simulink model "Comp_FDC_main"  (R2021b)
settings: Solver=FixedStepDiscrete  StartTime=0.0  StopTime=10.0  RelTol=1e-3  EnableMultiTasking=on
undefined symbols (not defined in the file or in its folder): D1, P
settings Model: DataDictionary=APPTypes.sldd  Creator=FVT23118  LastModifiedBy=FVT23118
settings SolverCC: AutoInsertRateTranBlk=on
settings DataIOCC: SaveFormat=StructureWithTime
settings OptimizationCC: DefaultParameterBehavior=Inlined  EnhancedBackFolding=on  PassReuseOutputArgsAs=Individual arguments  ZeroExternalMemoryAtStartup=off  ZeroInternalMemoryAtStartup=off  OptimizeBlockOrder=speed  DifferentSizesBufferReuse=on  OptimizationCustomize=off  EfficientTunableParamExpr=on
settings DebuggingCC: ParameterTunabilityLossMsg=error
settings ModelReferenceCC: ModelReferenceNumInstancesAllowed=Single
settings SFSimCC: MATLABDynamicMemAlloc=off
settings RTWCC: Description=AUTOSAR  SystemTargetFile=autosar.tlc  GenCodeOnly=on  TemplateMakefile=ert_default_tmf
settings CodeAppCC: ForceParamTrailComments=on  IgnoreCustomStorageClasses=off  OperatorAnnotations=on  SimulinkDataObjDesc=on  SFDataObjDesc=on  InsertBlockDesc=on
settings STFCustomTargetCC: TargetLangStandard=C99 (ISO)  MultiwordLength=256  ParMdlRefBuildCompliant=on  CompOptLevelCompliant=on  IncludeMdlTerminateFcn=off  CombineOutputUpdateFcns=on  SuppressErrorStatus=on  ERTCustomFileBanners=on  SupportNonFinite=off  SupportComplex=off  SupportContinuousTime=off  SupportNonInlinedSFcns=off  RemoveResetFunc=on  MATLABClassNameForMDSCustomization=Simulink.SoftwareTarget.ERTCustomization  AutosarCompliant=on  GRTInterface=off  UseToolchainInfoCompliant=on  LookupTableObjectStructAxisOrder=2,1,3,4,...  LUTObjectStructOrderEvenSpacing=Size,Table,Breakpoints  SystemTargetFile=autosar.tlc
settings ERTTargetCC: TargetLangStandard=C99 (ISO)  ConcurrentExecutionCompliant=off  IncludeMdlTerminateFcn=off  SuppressErrorStatus=on  SupportNonFinite=off  SupportComplex=off  ModelStepFunctionPrototypeControlCompliant=off  CPPClassGenCompliant=off  AutosarCompliant=on  LookupTableObjectStructAxisOrder=2,1,3,4,...  LUTObjectStructOrderEvenSpacing=Size,Table,Breakpoints  InlinedParameterPlacement=NonHierarchical  ERTCustomFileTemplate=example_file_process.tlc

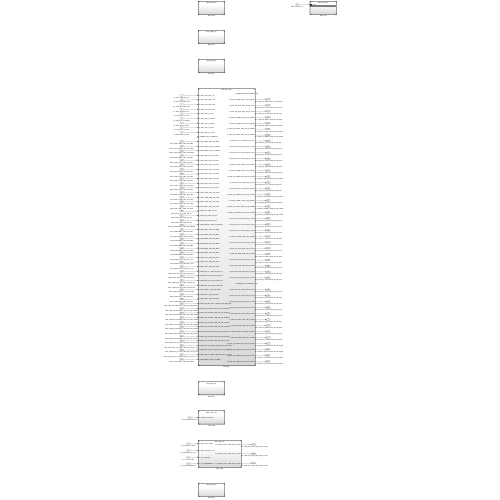
[thumbnail: Simulink's stored preview of the top-level diagram]
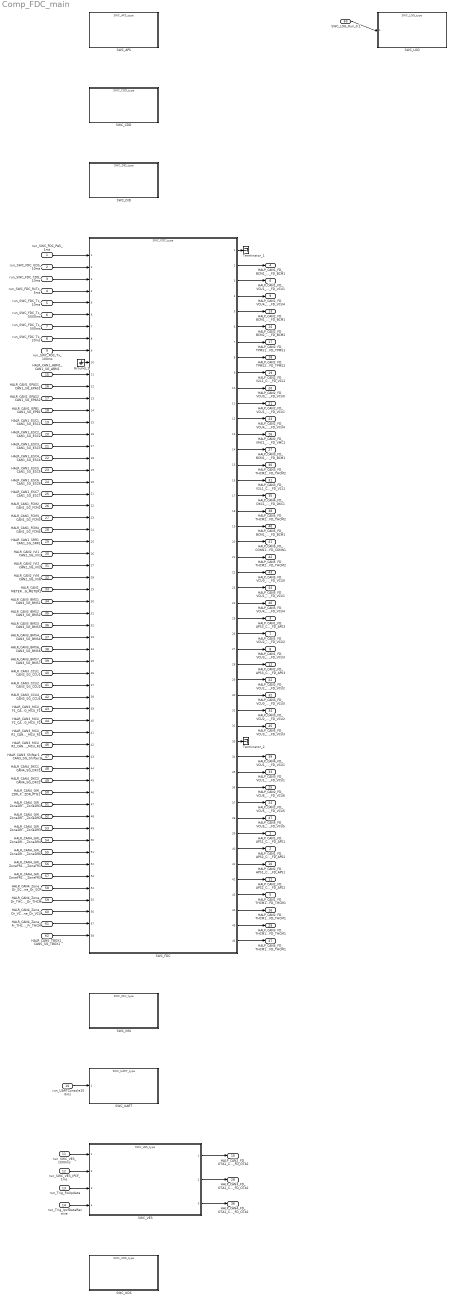
== system Comp_FDC_main ==
  run_SWC_FDC_PAS_1ms : Inport  SampleTime=0.001  OutputFunctionCall=on
  run_SWC_FDC_UDS_10ms : Inport  Port=2  SampleTime=0.01  OutputFunctionCall=on
  run_SWC_FDC_CDD_10ms : Inport  Port=3  SampleTime=0.01  OutputFunctionCall=on
  run_SWC_FDC_RxTx_5ms : Inport  Port=4  SampleTime=0.005  OutputFunctionCall=on
  run_SWC_FDC_Tx_10ms : Inport  Port=5  SampleTime=0.01  OutputFunctionCall=on
  run_SWC_FDC_Tx_5000ms : Inport  Port=6  SampleTime=5  OutputFunctionCall=on
  run_SWC_FDC_Tx_500ms : Inport  Port=7  SampleTime=0.5  OutputFunctionCall=on
  run_SWC_FDC_Tx_20ms : Inport  Port=8  SampleTime=0.02  OutputFunctionCall=on
  run_SWC_FDC_Tx_100ms : Inport  Port=9  SampleTime=0.1  OutputFunctionCall=on
  run_UARTConsole100ms : Inport  Port=10  SampleTime=0.1  OutputFunctionCall=on
  run_SWC_VES_1000ms : Inport  Port=11  SampleTime=1  OutputFunctionCall=on
  run_SWC_VES_IPCF_1ms : Inport  Port=12  SampleTime=0.001  OutputFunctionCall=on
  run_Trig_FwUpdate : Inport  Port=13  OutputFunctionCall=on
  run_Trig_IpcfDataReceive : Inport  Port=14  OutputFunctionCall=on
  HALR_CAN1_ABM1_CAN1_SG_ABM1 : Inport  Port=15  OutDataTypeStr=Bus: DT_CAN1_SG_ABM1  PortDimensions=1  BusOutputAsStruct=on
  HALR_CAN1_EPAS1_CAN1_SG_EPAS1 : Inport  Port=16  OutDataTypeStr=Bus: DT_CAN1_SG_EPAS1  PortDimensions=1  BusOutputAsStruct=on
  HALR_CAN1_EPAS2_CAN1_SG_EPAS2 : Inport  Port=17  OutDataTypeStr=Bus: DT_CAN1_SG_EPAS2  PortDimensions=1  BusOutputAsStruct=on
  HALR_CAN1_EPB1_CAN1_SG_EPB1 : Inport  Port=18  OutDataTypeStr=Bus: DT_CAN1_SG_EPB1  PortDimensions=1  BusOutputAsStruct=on
  HALR_CAN1_ESC1_CAN1_SG_ESC1 : Inport  Port=19  OutDataTypeStr=Bus: DT_CAN1_SG_ESC1  PortDimensions=1  BusOutputAsStruct=on
  HALR_CAN1_ESC2_CAN1_SG_ESC2 : Inport  Port=20  OutDataTypeStr=Bus: DT_CAN1_SG_ESC2  PortDimensions=1  BusOutputAsStruct=on
  HALR_CAN1_ESC3_CAN1_SG_ESC3 : Inport  Port=21  OutDataTypeStr=Bus: DT_CAN1_SG_ESC3  PortDimensions=1  BusOutputAsStruct=on
  HALR_CAN1_ESC4_CAN1_SG_ESC4 : Inport  Port=22  OutDataTypeStr=Bus: DT_CAN1_SG_ESC4  PortDimensions=1  BusOutputAsStruct=on
  HALR_CAN1_ESC5_CAN1_SG_ESC5 : Inport  Port=23  OutDataTypeStr=Bus: DT_CAN1_SG_ESC5  PortDimensions=1  BusOutputAsStruct=on
  HALR_CAN1_ESC6_CAN1_SG_ESC6 : Inport  Port=24  OutDataTypeStr=Bus: DT_CAN1_SG_ESC6  PortDimensions=1  BusOutputAsStruct=on
  HALR_CAN1_ESC7_CAN1_SG_ESC7 : Inport  Port=25  OutDataTypeStr=Bus: DT_CAN1_SG_ESC7  PortDimensions=1  BusOutputAsStruct=on
  HALR_CAN1_FCM2_CAN1_SG_FCM2 : Inport  Port=26  OutDataTypeStr=Bus: DT_CAN1_SG_FCM2  PortDimensions=1  BusOutputAsStruct=on
  HALR_CAN1_FCM3_CAN1_SG_FCM3 : Inport  Port=27  OutDataTypeStr=Bus: DT_CAN1_SG_FCM3  PortDimensions=1  BusOutputAsStruct=on
  HALR_CAN1_FCM4_CAN1_SG_FCM4 : Inport  Port=28  OutDataTypeStr=Bus: DT_CAN1_SG_FCM4  PortDimensions=1  BusOutputAsStruct=on
  HALR_CAN1_SRR1_CAN1_SG_SRR1 : Inport  Port=29  OutDataTypeStr=Bus: DT_CAN1_SG_SRR1  PortDimensions=1  BusOutputAsStruct=on
  HALR_CAN2_IVI1_CAN2_SG_IVI1 : Inport  Port=30  OutDataTypeStr=Bus: DT_CAN2_SG_IVI1  PortDimensions=1  BusOutputAsStruct=on
  HALR_CAN2_IVI2_CAN2_SG_IVI2 : Inport  Port=31  OutDataTypeStr=Bus: DT_CAN2_SG_IVI2  PortDimensions=1  BusOutputAsStruct=on
  HALR_CAN2_IVI6_CAN2_SG_IVI6 : Inport  Port=32  OutDataTypeStr=Bus: DT_CAN2_SG_IVI6  PortDimensions=1  BusOutputAsStruct=on
  HALR_CAN2_METER1_CAN2_SG_METER1 : Inport  Port=33  OutDataTypeStr=Bus: DT_CAN2_SG_METER1  PortDimensions=1  BusOutputAsStruct=on
  HALR_CAN3_BMS1_CAN3_SG_BMS1 : Inport  Port=34  OutDataTypeStr=Bus: DT_CAN3_SG_BMS1  PortDimensions=1  BusOutputAsStruct=on
  HALR_CAN3_BMS2_CAN3_SG_BMS2 : Inport  Port=35  OutDataTypeStr=Bus: DT_CAN3_SG_BMS2  PortDimensions=1  BusOutputAsStruct=on
  HALR_CAN3_BMS3_CAN3_SG_BMS3 : Inport  Port=36  OutDataTypeStr=Bus: DT_CAN3_SG_BMS3  PortDimensions=1  BusOutputAsStruct=on
  HALR_CAN3_BMS4_CAN3_SG_BMS4 : Inport  Port=37  OutDataTypeStr=Bus: DT_CAN3_SG_BMS4  PortDimensions=1  BusOutputAsStruct=on
  HALR_CAN3_BMS6_CAN3_SG_BMS6 : Inport  Port=38  OutDataTypeStr=Bus: DT_CAN3_SG_BMS6  PortDimensions=1  BusOutputAsStruct=on
  HALR_CAN3_BMS7_CAN3_SG_BMS7 : Inport  Port=39  OutDataTypeStr=Bus: DT_CAN3_SG_BMS7  PortDimensions=1  BusOutputAsStruct=on
  HALR_CAN3_CCU1_CAN3_SG_CCU1 : Inport  Port=40  OutDataTypeStr=Bus: DT_CAN3_SG_CCU1  PortDimensions=1  BusOutputAsStruct=on
  HALR_CAN3_CCU2_CAN3_SG_CCU2 : Inport  Port=41  OutDataTypeStr=Bus: DT_CAN3_SG_CCU2  PortDimensions=1  BusOutputAsStruct=on
  HALR_CAN3_CCU4_CAN3_SG_CCU4 : Inport  Port=42  OutDataTypeStr=Bus: DT_CAN3_SG_CCU4  PortDimensions=1  BusOutputAsStruct=on
  HALR_CAN3_MCU_F1_CAN3_SG_MCU_F1 : Inport  Port=43  OutDataTypeStr=Bus: DT_CAN3_SG_MCU_F1  PortDimensions=1  BusOutputAsStruct=on
  HALR_CAN3_MCU_F2_CAN3_SG_MCU_F2 : Inport  Port=44  OutDataTypeStr=Bus: DT_CAN3_SG_MCU_F2  PortDimensions=1  BusOutputAsStruct=on
  HALR_CAN3_MCU_R1_CAN3_SG_MCU_R1 : Inport  Port=45  OutDataTypeStr=Bus: DT_CAN3_SG_MCU_R1  PortDimensions=1  BusOutputAsStruct=on
  HALR_CAN3_MCU_R2_CAN3_SG_MCU_R2 : Inport  Port=46  OutDataTypeStr=Bus: DT_CAN3_SG_MCU_R2  PortDimensions=1  BusOutputAsStruct=on
  HALR_CAN3_Shifter1_CAN3_SG_Shifter1 : Inport  Port=47  OutDataTypeStr=Bus: DT_CAN3_SG_Shifter1  PortDimensions=1  BusOutputAsStruct=on
  HALR_CAN4_DKC1_CAN4_SG_DKC1 : Inport  Port=48  OutDataTypeStr=Bus: DT_CAN4_SG_DKC1  PortDimensions=1  BusOutputAsStruct=on
  HALR_CAN4_DKC2_CAN4_SG_DKC2 : Inport  Port=49  OutDataTypeStr=Bus: DT_CAN4_SG_DKC2  PortDimensions=1  BusOutputAsStruct=on
  HALR_CAN4_GW_ZDR_PTG1_CAN4_SG_GW_ZDR_PTG1 : Inport  Port=50  OutDataTypeStr=Bus: DT_CAN4_SG_GW_ZDR_PTG1  PortDimensions=1  BusOutputAsStruct=on
  HALR_CAN4_GW_ZoneDR1_CAN4_SG_GW_ZoneDR1 : Inport  Port=51  OutDataTypeStr=Bus: DT_CAN4_SG_GW_ZoneDR1  PortDimensions=1  BusOutputAsStruct=on
  HALR_CAN4_GW_ZoneDR2_CAN4_SG_GW_ZoneDR2 : Inport  Port=52  OutDataTypeStr=Bus: DT_CAN4_SG_GW_ZoneDR2  PortDimensions=1  BusOutputAsStruct=on
  HALR_CAN4_GW_ZoneDR3_CAN4_SG_GW_ZoneDR3 : Inport  Port=53  OutDataTypeStr=Bus: DT_CAN4_SG_GW_ZoneDR3  PortDimensions=1  BusOutputAsStruct=on
  HALR_CAN4_GW_ZoneDR4_CAN4_SG_GW_ZoneDR4 : Inport  Port=54  OutDataTypeStr=Bus: DT_CAN4_SG_GW_ZoneDR4  PortDimensions=1  BusOutputAsStruct=on
  HALR_CAN4_GW_ZoneDR6_CAN4_SG_GW_ZoneDR6 : Inport  Port=55  OutDataTypeStr=Bus: DT_CAN4_SG_GW_ZoneDR6  PortDimensions=1  BusOutputAsStruct=on
  HALR_CAN4_GW_ZoneFR1_CAN4_SG_GW_ZoneFR1 : Inport  Port=56  OutDataTypeStr=Bus: DT_CAN4_SG_GW_ZoneFR1  PortDimensions=1  BusOutputAsStruct=on
  HALR_CAN4_GW_ZoneFR2_CAN4_SG_GW_ZoneFR2 : Inport  Port=57  OutDataTypeStr=Bus: DT_CAN4_SG_GW_ZoneFR2  PortDimensions=1  BusOutputAsStruct=on
  HALR_CAN4_Zone_Dr_SCP_CAN4_SG_Zone_Dr_SCP : Inport  Port=58  OutDataTypeStr=Bus: DT_CAN4_SG_Zone_Dr_SCP  PortDimensions=1  BusOutputAsStruct=on
  HALR_CAN4_Zone_Dr_THCM_CAN4_SG_Zone_Dr_THCM : Inport  Port=59  OutDataTypeStr=Bus: DT_CAN4_SG_Zone_Dr_THCM  PortDimensions=1  BusOutputAsStruct=on
  HALR_CAN4_Zone_Dr_VCU_CAN4_SG_Zone_Dr_VCU : Inport  Port=60  OutDataTypeStr=Bus: DT_CAN4_SG_Zone_Dr_VCU  PortDimensions=1  BusOutputAsStruct=on
  HALR_CAN4_Zone_Fr_THCM_CAN4_SG_Zone_Fr_THCM : Inport  Port=61  OutDataTypeStr=Bus: DT_CAN4_SG_Zone_Fr_THCM  PortDimensions=1  BusOutputAsStruct=on
  HALR_CAN5_TBOX1_CAN5_SG_TBOX1 : Inport  Port=62  OutDataTypeStr=Bus: DT_CAN5_SG_TBOX1  PortDimensions=1  BusOutputAsStruct=on
  SWC_LOG_Run_0.1 : Inport  Port=63  SampleTime=0.1  OutputFunctionCall=on
  Ground_1 : Ground
  SWC_APS : ModelReference  ModelNameDialog=SWC_APS_type  SimulationMode=Normal  ScheduleRates=on  ModelReferenceVersion=1.3
  SWC_CDD : ModelReference  ModelNameDialog=SWC_CDD_type  SimulationMode=Normal  ScheduleRates=on  ModelReferenceVersion=1.5
  SWC_DID : ModelReference  ModelNameDialog=SWC_DID_type  SimulationMode=Normal  ScheduleRates=on  ModelReferenceVersion=1.5
  SWC_FDC : ModelReference  ModelNameDialog=SWC_FDC_type  SimulationMode=Normal  ScheduleRates=on  ModelReferenceVersion=1.30
  SWC_IMU : ModelReference  ModelNameDialog=SWC_IMU_type  SimulationMode=Normal  ScheduleRates=on  ModelReferenceVersion=1.3
  SWC_LOG : ModelReference  ModelNameDialog=SWC_LOG_type  SimulationMode=Normal  ScheduleRates=on  PortDiscreteRates=[0.1]  CachedPortDiscreteRates=[0.1]  ModelEventPortInfo=P:D1[0.1][0][0]  ModelReferenceVersion=1.4
  SWC_UART : ModelReference  ModelNameDialog=SWC_UART_type  SimulationMode=Normal  ScheduleRates=on  ModelReferenceVersion=1.3
  SWC_UDS : ModelReference  ModelNameDialog=SWC_UDS_type  SimulationMode=Normal  ScheduleRates=on  ModelReferenceVersion=1.3
  SWC_VES : ModelReference  ModelNameDialog=SWC_VES_type  SimulationMode=Normal  ScheduleRates=on  ModelReferenceVersion=1.4
  Terminator_1 : Terminator
  Terminator_2 : Terminator
  HALP_CAN1_FD_APS1_CAN1_SG_FD_APS1 : Outport  OutDataTypeStr=Bus: DT_CAN1_SG_FD_APS1  PortDimensions=1  BusOutputAsStruct=on
  HALP_CAN1_FD_APS2_CAN1_SG_FD_APS2 : Outport  Port=2  OutDataTypeStr=Bus: DT_CAN1_SG_FD_APS2  PortDimensions=1  BusOutputAsStruct=on
  HALP_CAN1_FD_APS3_CAN1_SG_FD_APS3 : Outport  Port=3  OutDataTypeStr=Bus: DT_CAN1_SG_FD_APS3  PortDimensions=1  BusOutputAsStruct=on
  HALP_CAN1_FD_BCM1_CAN1_SG_FD_BCM1 : Outport  Port=4  OutDataTypeStr=Bus: DT_CAN1_SG_FD_BCM1  PortDimensions=1  BusOutputAsStruct=on
  HALP_CAN1_FD_THCM1_CAN1_SG_FD_THCM1 : Outport  Port=5  OutDataTypeStr=Bus: DT_CAN1_SG_FD_THCM1  PortDimensions=1  BusOutputAsStruct=on
  HALP_CAN1_FD_VCU1_CAN1_SG_FD_VCU1 : Outport  Port=6  OutDataTypeStr=Bus: DT_CAN1_SG_FD_VCU1  PortDimensions=1  BusOutputAsStruct=on
  HALP_CAN1_FD_VCU2_CAN1_SG_FD_VCU2 : Outport  Port=7  OutDataTypeStr=Bus: DT_CAN1_SG_FD_VCU2  PortDimensions=1  BusOutputAsStruct=on
  HALP_CAN1_FD_VCU3_CAN1_SG_FD_VCU3 : Outport  Port=8  OutDataTypeStr=Bus: DT_CAN1_SG_FD_VCU3  PortDimensions=1  BusOutputAsStruct=on
  HALP_CAN1_FD_VCU4_CAN1_SG_FD_VCU4 : Outport  Port=9  OutDataTypeStr=Bus: DT_CAN1_SG_FD_VCU4  PortDimensions=1  BusOutputAsStruct=on
  HALP_CAN2_FD_APS1_CAN2_SG_FD_APS1 : Outport  Port=10  OutDataTypeStr=Bus: DT_CAN2_SG_FD_APS1  PortDimensions=1  BusOutputAsStruct=on
  HALP_CAN2_FD_APS2_CAN2_SG_FD_APS2 : Outport  Port=11  OutDataTypeStr=Bus: DT_CAN2_SG_FD_APS2  PortDimensions=1  BusOutputAsStruct=on
  HALP_CAN2_FD_APS3_CAN2_SG_FD_APS3 : Outport  Port=12  OutDataTypeStr=Bus: DT_CAN2_SG_FD_APS3  PortDimensions=1  BusOutputAsStruct=on
  HALP_CAN2_FD_BCM1_CAN2_SG_FD_BCM1 : Outport  Port=13  OutDataTypeStr=Bus: DT_CAN2_SG_FD_BCM1  PortDimensions=1  BusOutputAsStruct=on
  HALP_CAN2_FD_BCM2_CAN2_SG_FD_BCM2 : Outport  Port=14  OutDataTypeStr=Bus: DT_CAN2_SG_FD_BCM2  PortDimensions=1  BusOutputAsStruct=on
  HALP_CAN2_FD_OTA1_CAN2_SG_FD_OTA1 : Outport  Port=15  OutDataTypeStr=Bus: DT_CAN2_SG_FD_OTA1  PortDimensions=1  BusOutputAsStruct=on
  HALP_CAN2_FD_THCM1_CAN2_SG_FD_THCM1 : Outport  Port=16  OutDataTypeStr=Bus: DT_CAN2_SG_FD_THCM1  PortDimensions=1  BusOutputAsStruct=on
  HALP_CAN2_FD_TPMS1_CAN2_SG_FD_TPMS1 : Outport  Port=17  OutDataTypeStr=Bus: DT_CAN2_SG_FD_TPMS1  PortDimensions=1  BusOutputAsStruct=on
  HALP_CAN2_FD_TPMS2_CAN2_SG_FD_TPMS2 : Outport  Port=18  OutDataTypeStr=Bus: DT_CAN2_SG_FD_TPMS2  PortDimensions=1  BusOutputAsStruct=on
  HALP_CAN2_FD_V2L1_CAN2_SG_FD_V2L1 : Outport  Port=19  OutDataTypeStr=Bus: DT_CAN2_SG_FD_V2L1  PortDimensions=1  BusOutputAsStruct=on
  HALP_CAN2_FD_VCU0_CAN2_SG_FD_VCU0 : Outport  Port=20  OutDataTypeStr=Bus: DT_CAN2_SG_FD_VCU0  PortDimensions=1  BusOutputAsStruct=on
  HALP_CAN2_FD_VCU1_CAN2_SG_FD_VCU1 : Outport  Port=21  OutDataTypeStr=Bus: DT_CAN2_SG_FD_VCU1  PortDimensions=1  BusOutputAsStruct=on
  HALP_CAN2_FD_VCU2_CAN2_SG_FD_VCU2 : Outport  Port=22  OutDataTypeStr=Bus: DT_CAN2_SG_FD_VCU2  PortDimensions=1  BusOutputAsStruct=on
  HALP_CAN2_FD_VCU4_CAN2_SG_FD_VCU4 : Outport  Port=23  OutDataTypeStr=Bus: DT_CAN2_SG_FD_VCU4  PortDimensions=1  BusOutputAsStruct=on
  HALP_CAN2_FD_VCU5_CAN2_SG_FD_VCU5 : Outport  Port=24  OutDataTypeStr=Bus: DT_CAN2_SG_FD_VCU5  PortDimensions=1  BusOutputAsStruct=on
  HALP_CAN2_FD_VCU6_CAN2_SG_FD_VCU6 : Outport  Port=25  OutDataTypeStr=Bus: DT_CAN2_SG_FD_VCU6  PortDimensions=1  BusOutputAsStruct=on
  HALP_CAN2_FD_VMC1_CAN2_SG_FD_VMC1 : Outport  Port=26  OutDataTypeStr=Bus: DT_CAN2_SG_FD_VMC1  PortDimensions=1  BusOutputAsStruct=on
  HALP_CAN3_FD_BCM1_CAN3_SG_FD_BCM1 : Outport  Port=27  OutDataTypeStr=Bus: DT_CAN3_SG_FD_BCM1  PortDimensions=1  BusOutputAsStruct=on
  HALP_CAN3_FD_OTA1_CAN3_SG_FD_OTA1 : Outport  Port=28  OutDataTypeStr=Bus: DT_CAN3_SG_FD_OTA1  PortDimensions=1  BusOutputAsStruct=on
  HALP_CAN3_FD_THCM1_CAN3_SG_FD_THCM1 : Outport  Port=29  OutDataTypeStr=Bus: DT_CAN3_SG_FD_THCM1  PortDimensions=1  BusOutputAsStruct=on
  HALP_CAN3_FD_THCM2_CAN3_SG_FD_THCM2 : Outport  Port=30  OutDataTypeStr=Bus: DT_CAN3_SG_FD_THCM2  PortDimensions=1  BusOutputAsStruct=on
  HALP_CAN3_FD_V2L1_CAN3_SG_FD_V2L1 : Outport  Port=31  OutDataTypeStr=Bus: DT_CAN3_SG_FD_V2L1  PortDimensions=1  BusOutputAsStruct=on
  HALP_CAN3_FD_VCU0_CAN3_SG_FD_VCU0 : Outport  Port=32  OutDataTypeStr=Bus: DT_CAN3_SG_FD_VCU0  PortDimensions=1  BusOutputAsStruct=on
  HALP_CAN3_FD_VCU1_CAN3_SG_FD_VCU1 : Outport  Port=33  OutDataTypeStr=Bus: DT_CAN3_SG_FD_VCU1  PortDimensions=1  BusOutputAsStruct=on
  HALP_CAN3_FD_VCU2_CAN3_SG_FD_VCU2 : Outport  Port=34  OutDataTypeStr=Bus: DT_CAN3_SG_FD_VCU2  PortDimensions=1  BusOutputAsStruct=on
  HALP_CAN4_FD_DKC1_CAN4_SG_FD_DKC1 : Outport  Port=35  OutDataTypeStr=Bus: DT_CAN4_SG_FD_DKC1  PortDimensions=1  BusOutputAsStruct=on
  HALP_CAN4_FD_OTA1_CAN4_SG_FD_OTA1 : Outport  Port=36  OutDataTypeStr=Bus: DT_CAN4_SG_FD_OTA1  PortDimensions=1  BusOutputAsStruct=on
  HALP_CAN4_FD_THCM1_CAN4_SG_FD_THCM1 : Outport  Port=37  OutDataTypeStr=Bus: DT_CAN4_SG_FD_THCM1  PortDimensions=1  BusOutputAsStruct=on
  HALP_CAN4_FD_THCM2_CAN4_SG_FD_THCM2 : Outport  Port=38  OutDataTypeStr=Bus: DT_CAN4_SG_FD_THCM2  PortDimensions=1  BusOutputAsStruct=on
  HALP_CAN4_FD_VCU1_CAN4_SG_FD_VCU1 : Outport  Port=39  OutDataTypeStr=Bus: DT_CAN4_SG_FD_VCU1  PortDimensions=1  BusOutputAsStruct=on
  HALP_CAN5_FD_BCM1_CAN5_SG_FD_BCM1 : Outport  Port=40  OutDataTypeStr=Bus: DT_CAN5_SG_FD_BCM1  PortDimensions=1  BusOutputAsStruct=on
  HALP_CAN5_FD_CONN1_CAN5_SG_FD_CONN1 : Outport  Port=41  OutDataTypeStr=Bus: DT_CAN5_SG_FD_CONN1  PortDimensions=1  BusOutputAsStruct=on
  HALP_CAN5_FD_THCM2_CAN5_SG_FD_THCM2 : Outport  Port=42  OutDataTypeStr=Bus: DT_CAN5_SG_FD_THCM2  PortDimensions=1  BusOutputAsStruct=on
  HALP_CAN5_FD_VCU0_CAN5_SG_FD_VCU0 : Outport  Port=43  OutDataTypeStr=Bus: DT_CAN5_SG_FD_VCU0  PortDimensions=1  BusOutputAsStruct=on
  HALP_CAN5_FD_VCU1_CAN5_SG_FD_VCU1 : Outport  Port=44  OutDataTypeStr=Bus: DT_CAN5_SG_FD_VCU1  PortDimensions=1  BusOutputAsStruct=on
  HALP_CAN5_FD_VCU3_CAN5_SG_FD_VCU3 : Outport  Port=45  OutDataTypeStr=Bus: DT_CAN5_SG_FD_VCU3  PortDimensions=1  BusOutputAsStruct=on
  HALP_CAN5_FD_VCU4_CAN5_SG_FD_VCU4 : Outport  Port=46  OutDataTypeStr=Bus: DT_CAN5_SG_FD_VCU4  PortDimensions=1  BusOutputAsStruct=on
  HALP_CAN5_FD_VCU5_CAN5_SG_FD_VCU5 : Outport  Port=47  OutDataTypeStr=Bus: DT_CAN5_SG_FD_VCU5  PortDimensions=1  BusOutputAsStruct=on
  wires:
  run_SWC_FDC_PAS_1ms/1 -> SWC_FDC/1
  run_SWC_FDC_UDS_10ms/1 -> SWC_FDC/2
  run_SWC_FDC_CDD_10ms/1 -> SWC_FDC/3
  run_SWC_FDC_RxTx_5ms/1 -> SWC_FDC/4
  run_SWC_FDC_Tx_10ms/1 -> SWC_FDC/5
  run_SWC_FDC_Tx_5000ms/1 -> SWC_FDC/6
  run_SWC_FDC_Tx_500ms/1 -> SWC_FDC/7
  run_SWC_FDC_Tx_20ms/1 -> SWC_FDC/8
  run_SWC_FDC_Tx_100ms/1 -> SWC_FDC/9
  run_UARTConsole100ms/1 -> SWC_UART/1
  run_SWC_VES_1000ms/1 -> SWC_VES/1
  run_SWC_VES_IPCF_1ms/1 -> SWC_VES/2
  run_Trig_FwUpdate/1 -> SWC_VES/3
  run_Trig_IpcfDataReceive/1 -> SWC_VES/4
  HALR_CAN1_ABM1_CAN1_SG_ABM1/1 -> SWC_FDC/11
  HALR_CAN1_EPAS1_CAN1_SG_EPAS1/1 -> SWC_FDC/12
  HALR_CAN1_EPAS2_CAN1_SG_EPAS2/1 -> SWC_FDC/13
  HALR_CAN1_EPB1_CAN1_SG_EPB1/1 -> SWC_FDC/14
  HALR_CAN1_ESC1_CAN1_SG_ESC1/1 -> SWC_FDC/15
  HALR_CAN1_ESC2_CAN1_SG_ESC2/1 -> SWC_FDC/16
  HALR_CAN1_ESC3_CAN1_SG_ESC3/1 -> SWC_FDC/17
  HALR_CAN1_ESC4_CAN1_SG_ESC4/1 -> SWC_FDC/18
  HALR_CAN1_ESC5_CAN1_SG_ESC5/1 -> SWC_FDC/19
  HALR_CAN1_ESC6_CAN1_SG_ESC6/1 -> SWC_FDC/20
  HALR_CAN1_ESC7_CAN1_SG_ESC7/1 -> SWC_FDC/21
  HALR_CAN1_FCM2_CAN1_SG_FCM2/1 -> SWC_FDC/22
  HALR_CAN1_FCM3_CAN1_SG_FCM3/1 -> SWC_FDC/23
  HALR_CAN1_FCM4_CAN1_SG_FCM4/1 -> SWC_FDC/24
  HALR_CAN1_SRR1_CAN1_SG_SRR1/1 -> SWC_FDC/25
  HALR_CAN2_IVI1_CAN2_SG_IVI1/1 -> SWC_FDC/26
  HALR_CAN2_IVI2_CAN2_SG_IVI2/1 -> SWC_FDC/27
  HALR_CAN2_IVI6_CAN2_SG_IVI6/1 -> SWC_FDC/28
  HALR_CAN2_METER1_CAN2_SG_METER1/1 -> SWC_FDC/29
  HALR_CAN3_BMS1_CAN3_SG_BMS1/1 -> SWC_FDC/30
  HALR_CAN3_BMS2_CAN3_SG_BMS2/1 -> SWC_FDC/31
  HALR_CAN3_BMS3_CAN3_SG_BMS3/1 -> SWC_FDC/32
  HALR_CAN3_BMS4_CAN3_SG_BMS4/1 -> SWC_FDC/33
  HALR_CAN3_BMS6_CAN3_SG_BMS6/1 -> SWC_FDC/34
  HALR_CAN3_BMS7_CAN3_SG_BMS7/1 -> SWC_FDC/35
  HALR_CAN3_CCU1_CAN3_SG_CCU1/1 -> SWC_FDC/36
  HALR_CAN3_CCU2_CAN3_SG_CCU2/1 -> SWC_FDC/37
  HALR_CAN3_CCU4_CAN3_SG_CCU4/1 -> SWC_FDC/38
  HALR_CAN3_MCU_F1_CAN3_SG_MCU_F1/1 -> SWC_FDC/39
  HALR_CAN3_MCU_F2_CAN3_SG_MCU_F2/1 -> SWC_FDC/40
  HALR_CAN3_MCU_R1_CAN3_SG_MCU_R1/1 -> SWC_FDC/41
  HALR_CAN3_MCU_R2_CAN3_SG_MCU_R2/1 -> SWC_FDC/42
  HALR_CAN3_Shifter1_CAN3_SG_Shifter1/1 -> SWC_FDC/43
  HALR_CAN4_DKC1_CAN4_SG_DKC1/1 -> SWC_FDC/44
  HALR_CAN4_DKC2_CAN4_SG_DKC2/1 -> SWC_FDC/45
  HALR_CAN4_GW_ZDR_PTG1_CAN4_SG_GW_ZDR_PTG1/1 -> SWC_FDC/46
  HALR_CAN4_GW_ZoneDR1_CAN4_SG_GW_ZoneDR1/1 -> SWC_FDC/47
  HALR_CAN4_GW_ZoneDR2_CAN4_SG_GW_ZoneDR2/1 -> SWC_FDC/48
  HALR_CAN4_GW_ZoneDR3_CAN4_SG_GW_ZoneDR3/1 -> SWC_FDC/49
  HALR_CAN4_GW_ZoneDR4_CAN4_SG_GW_ZoneDR4/1 -> SWC_FDC/50
  HALR_CAN4_GW_ZoneDR6_CAN4_SG_GW_ZoneDR6/1 -> SWC_FDC/51
  HALR_CAN4_GW_ZoneFR1_CAN4_SG_GW_ZoneFR1/1 -> SWC_FDC/52
  HALR_CAN4_GW_ZoneFR2_CAN4_SG_GW_ZoneFR2/1 -> SWC_FDC/53
  HALR_CAN4_Zone_Dr_SCP_CAN4_SG_Zone_Dr_SCP/1 -> SWC_FDC/54
  HALR_CAN4_Zone_Dr_THCM_CAN4_SG_Zone_Dr_THCM/1 -> SWC_FDC/55
  HALR_CAN4_Zone_Dr_VCU_CAN4_SG_Zone_Dr_VCU/1 -> SWC_FDC/56
  HALR_CAN4_Zone_Fr_THCM_CAN4_SG_Zone_Fr_THCM/1 -> SWC_FDC/57
  HALR_CAN5_TBOX1_CAN5_SG_TBOX1/1 -> SWC_FDC/58
  SWC_FDC/39 -> HALP_CAN1_FD_APS1_CAN1_SG_FD_APS1/1
  SWC_FDC/40 -> HALP_CAN1_FD_APS2_CAN1_SG_FD_APS2/1
  SWC_FDC/25 -> HALP_CAN1_FD_APS3_CAN1_SG_FD_APS3/1
  SWC_FDC/2 -> HALP_CAN1_FD_BCM1_CAN1_SG_FD_BCM1/1
  SWC_FDC/43 -> HALP_CAN1_FD_THCM1_CAN1_SG_FD_THCM1/1
  SWC_FDC/3 -> HALP_CAN1_FD_VCU1_CAN1_SG_FD_VCU1/1
  SWC_FDC/26 -> HALP_CAN1_FD_VCU2_CAN1_SG_FD_VCU2/1
  SWC_FDC/27 -> HALP_CAN1_FD_VCU3_CAN1_SG_FD_VCU3/1
  SWC_FDC/4 -> HALP_CAN1_FD_VCU4_CAN1_SG_FD_VCU4/1
  SWC_FDC/41 -> HALP_CAN2_FD_APS1_CAN2_SG_FD_APS1/1
  SWC_FDC/42 -> HALP_CAN2_FD_APS2_CAN2_SG_FD_APS2/1
  SWC_FDC/28 -> HALP_CAN2_FD_APS3_CAN2_SG_FD_APS3/1
  SWC_FDC/5 -> HALP_CAN2_FD_BCM1_CAN2_SG_FD_BCM1/1
  SWC_FDC/6 -> HALP_CAN2_FD_BCM2_CAN2_SG_FD_BCM2/1
  SWC_VES/1 -> HALP_CAN2_FD_OTA1_CAN2_SG_FD_OTA1/1
  SWC_FDC/44 -> HALP_CAN2_FD_THCM1_CAN2_SG_FD_THCM1/1
  SWC_FDC/7 -> HALP_CAN2_FD_TPMS1_CAN2_SG_FD_TPMS1/1
  SWC_FDC/8 -> HALP_CAN2_FD_TPMS2_CAN2_SG_FD_TPMS2/1
  SWC_FDC/9 -> HALP_CAN2_FD_V2L1_CAN2_SG_FD_V2L1/1
  SWC_FDC/10 -> HALP_CAN2_FD_VCU0_CAN2_SG_FD_VCU0/1
  SWC_FDC/11 -> HALP_CAN2_FD_VCU1_CAN2_SG_FD_VCU1/1
  SWC_FDC/29 -> HALP_CAN2_FD_VCU2_CAN2_SG_FD_VCU2/1
  SWC_FDC/12 -> HALP_CAN2_FD_VCU4_CAN2_SG_FD_VCU4/1
  SWC_FDC/37 -> HALP_CAN2_FD_VCU5_CAN2_SG_FD_VCU5/1
  SWC_FDC/36 -> HALP_CAN2_FD_VCU6_CAN2_SG_FD_VCU6/1
  SWC_FDC/13 -> HALP_CAN2_FD_VMC1_CAN2_SG_FD_VMC1/1
  SWC_FDC/14 -> HALP_CAN3_FD_BCM1_CAN3_SG_FD_BCM1/1
  SWC_VES/2 -> HALP_CAN3_FD_OTA1_CAN3_SG_FD_OTA1/1
  SWC_FDC/45 -> HALP_CAN3_FD_THCM1_CAN3_SG_FD_THCM1/1
  SWC_FDC/15 -> HALP_CAN3_FD_THCM2_CAN3_SG_FD_THCM2/1
  SWC_FDC/16 -> HALP_CAN3_FD_V2L1_CAN3_SG_FD_V2L1/1
  SWC_FDC/30 -> HALP_CAN3_FD_VCU0_CAN3_SG_FD_VCU0/1
  SWC_FDC/35 -> HALP_CAN3_FD_VCU1_CAN3_SG_FD_VCU1/1
  SWC_FDC/31 -> HALP_CAN3_FD_VCU2_CAN3_SG_FD_VCU2/1
  SWC_FDC/17 -> HALP_CAN4_FD_DKC1_CAN4_SG_FD_DKC1/1
  SWC_VES/3 -> HALP_CAN4_FD_OTA1_CAN4_SG_FD_OTA1/1
  SWC_FDC/46 -> HALP_CAN4_FD_THCM1_CAN4_SG_FD_THCM1/1
  SWC_FDC/18 -> HALP_CAN4_FD_THCM2_CAN4_SG_FD_THCM2/1
  SWC_FDC/34 -> HALP_CAN4_FD_VCU1_CAN4_SG_FD_VCU1/1
  SWC_FDC/19 -> HALP_CAN5_FD_BCM1_CAN5_SG_FD_BCM1/1
  SWC_FDC/20 -> HALP_CAN5_FD_CONN1_CAN5_SG_FD_CONN1/1
  SWC_FDC/21 -> HALP_CAN5_FD_THCM2_CAN5_SG_FD_THCM2/1
  SWC_FDC/22 -> HALP_CAN5_FD_VCU0_CAN5_SG_FD_VCU0/1
  SWC_FDC/23 -> HALP_CAN5_FD_VCU1_CAN5_SG_FD_VCU1/1
  SWC_FDC/32 -> HALP_CAN5_FD_VCU3_CAN5_SG_FD_VCU3/1
  SWC_FDC/24 -> HALP_CAN5_FD_VCU4_CAN5_SG_FD_VCU4/1
  SWC_FDC/38 -> HALP_CAN5_FD_VCU5_CAN5_SG_FD_VCU5/1
  Ground_1/1 -> SWC_FDC/10
  SWC_FDC/1 -> Terminator_1/1
  SWC_FDC/33 -> Terminator_2/1
  SWC_LOG_Run_0.1/1 -> SWC_LOG/1
